simulink model "verify_Pipe_stratified_charge_mdl"  (R2016b)
settings: Solver=VariableStepDiscrete  StartTime=0  StopTime=10  MaxStep=1  RelTol=1e-3  EnableMultiTasking=on
InitFcn:
  | height =1.47;
  | dia = 0.525;
  | nodes = 5;
libraries: carnot x2, simulink x2
settings Model: Creator=drhf  LastModifiedBy=drhf
settings DataIOCC: SaveFormat=Array  SignalLoggingSaveFormat=ModelDataLogs
settings OptimizationCC: ExpressionDepthLimit=2147483647  LifeSpan=inf
settings DebuggingCC: UnderspecifiedInitializationDetection=Classic  MergeDetectMultiDrivingBlocksExec=none  SolverPrmCheckMsg=warning  FcnCallInpInsideContextMsg=warning  StateNameClashWarn=warning  SFUnexpectedBacktrackingDiag=warning  SFNoUnconditionalDefaultTransitionDiag=warning  SFExecutionAtInitializationDiag=none
settings HardwareCC: ProdBitPerPointer=32  ProdBitPerSizeT=32  ProdBitPerPtrDiffT=32  ProdLargestAtomicFloat=None  ProdIntDivRoundTo=Undefined  ProdEndianess=Unspecified  ProdWordSize=32  ProdHWDeviceType=32-bit Generic
settings ModelReferenceCC: PropagateSignalLabelsOutOfModel=off
settings GRTTargetCC: TargetLangStandard=C89/C90 (ANSI)  GeneratePreprocessorConditionals=Disable all  CombineOutputUpdateFcns=off  GRTInterface=on
settings ConfigComp: CovMetricSettings=dw  CovHtmlReporting=on  CovSaveCumulativeToWorkspaceVar=on  CovSaveSingleToWorkspaceVar=on  CovExternalEMLEnable=off

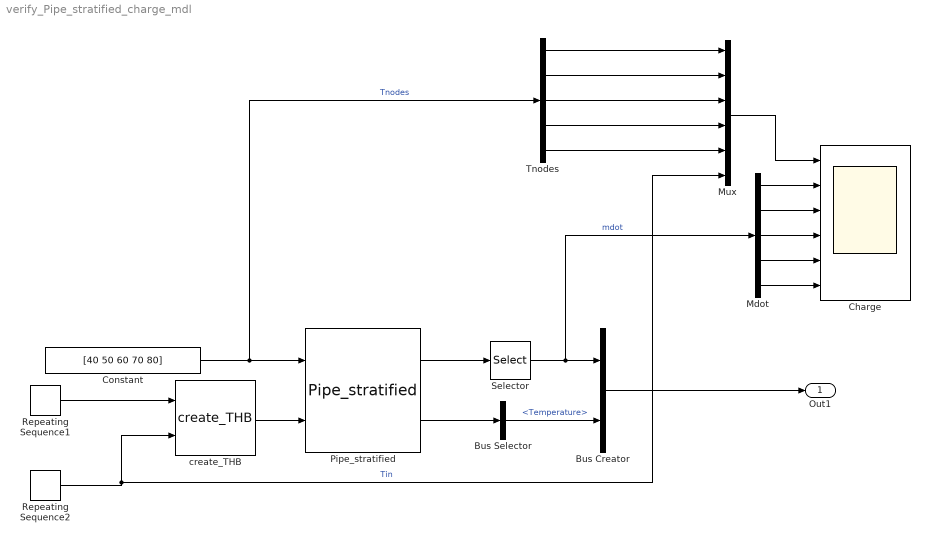
== system verify_Pipe_stratified_charge_mdl ==
  Bus Creator : BusCreator  Inputs=2
  Bus Selector : BusSelector  OutputSignals=Temperature
  Charge : Scope  NumInputPorts=6
  Constant : Constant  Value=[40 50 60 70 80]
  Mdot : Demux  Outputs=5
  Mux : Mux  Inputs=6
  Pipe_stratified : carnot/Storage/Thermal/Storage_Ports/Pipe_stratified  h_in=0.9  h_out=0.1  hgt=1  dia=0.02  height=-0.8  nodes=nodes
  Repeating Sequence1 : simulink/Sources/Repeating Sequence  rep_seq_t=[0 5 10]  rep_seq_y=[100/3600 500/3600 100/3600]
  Repeating Sequence2 : simulink/Sources/Repeating Sequence  rep_seq_t=[0 5 10]  rep_seq_y=[30 90 30]
  Selector : Selector  InputPortWidth=28  IndexOptions=Index vector (dialog)  Indices=[6:10]  OutputSizes=1
  Tnodes : Demux  Outputs=5
  create_THB : carnot/Source/Simple/create_THB  p=1e5  fluid=Water  mix=0  mix2=0  mix3=0  dia=0.02  hgt=0  mID=No Pressure Drop
  Out1 : Outport
  wires:
  Pipe_stratified/1 -> Selector/1
  Pipe_stratified/2 -> Bus Selector/1
  Selector/1 -> Mdot/1, Bus Creator/1  "mdot"
  Bus Selector/1 -> Bus Creator/2  "<Temperature>"
  Bus Creator/1 -> Out1/1
  Constant/1 -> Tnodes/1, Pipe_stratified/1  "Tnodes"
  create_THB/1 -> Pipe_stratified/2
  Repeating Sequence1/1 -> create_THB/1
  Repeating Sequence2/1 -> Mux/6, create_THB/2  "Tin"
  Mux/1 -> Charge/1
  Mdot/3 -> Charge/4
  Mdot/2 -> Charge/3
  Mdot/4 -> Charge/5
  Mdot/5 -> Charge/6
  Mdot/1 -> Charge/2
  Tnodes/4 -> Mux/4
  Tnodes/1 -> Mux/1
  Tnodes/3 -> Mux/3
  Tnodes/2 -> Mux/2
  Tnodes/5 -> Mux/5
